simulink model "LinearSimulation"  (R2022b)
settings: Solver=VariableStepAuto  StartTime=0.0  StopTime=10  RelTol=1e-3
undefined symbols (not defined in the file): K, L, T
settings Model: Creator=amirz  LastModifiedBy=amirz

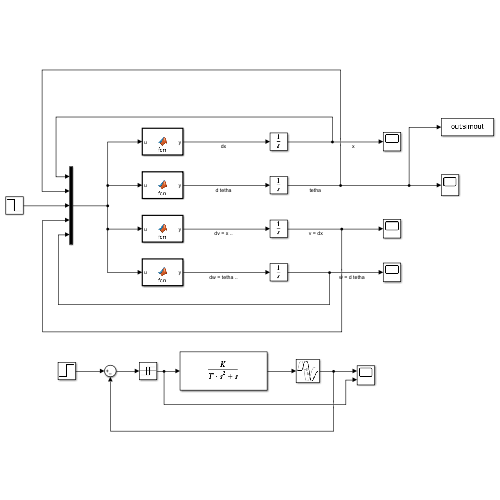
[thumbnail: Simulink's stored preview of the top-level diagram]
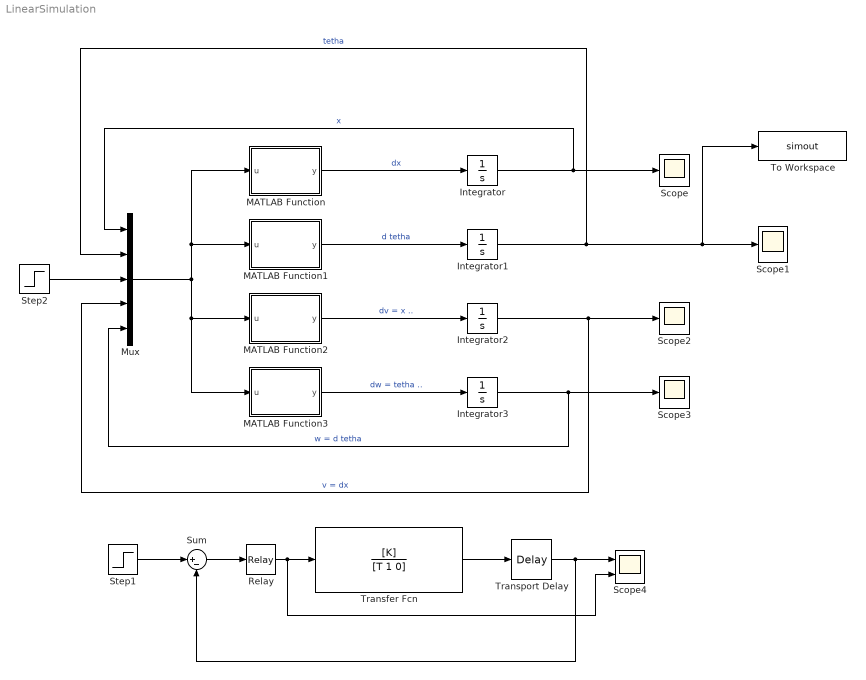
== system LinearSimulation ==
  Integrator{,1..3} (4 alike) : Integrator
  MATLAB Function : MATLAB Function  TreatAsAtomicUnit=on
  MATLAB Function1 : MATLAB Function  TreatAsAtomicUnit=on
  MATLAB Function2 : MATLAB Function  TreatAsAtomicUnit=on
  MATLAB Function3 : MATLAB Function  TreatAsAtomicUnit=on
  Mux : Mux  Inputs=5
  Relay : Relay  OffOutputValue=-1
  Scope{,1..3} (4 alike) : Scope
  Scope4 : Scope  NumInputPorts=2
  Step1 : Step  Time=0  After=0  SampleTime=0
  Step2 : Step  Time=0  After=-1  SampleTime=0
  Sum : Sum  Inputs=|+-
  To Workspace : ToWorkspace  VariableName=simout  SaveFormat=Timeseries  SampleTime=-1
  Transfer Fcn : TransferFcn  Numerator=[K]  Denominator=[T 1 0]
  Transport Delay : TransportDelay  DelayTime=L
  wires:
  Mux/1 -> MATLAB Function2/1(u), MATLAB Function3/1(u), MATLAB Function/1(u), MATLAB Function1/1(u)
  Integrator2/1 -> Scope2/1, Mux/4  "v = dx"
  MATLAB Function1/1(y) -> Integrator1/1  "d tetha"
  MATLAB Function/1(y) -> Integrator/1  "dx"
  Integrator1/1 -> To Workspace/1, Scope1/1, Mux/2  "tetha"
  MATLAB Function2/1(y) -> Integrator2/1  "dv = x .."
  Integrator/1 -> Mux/1, Scope/1  "x"
  MATLAB Function3/1(y) -> Integrator3/1  "dw = tetha .."
  Integrator3/1 -> Mux/5, Scope3/1  "w = d tetha"
  Step2/1 -> Mux/3
  Transfer Fcn/1 -> Transport Delay/1
  Transport Delay/1 -> Scope4/1, Sum/2
  Relay/1 -> Scope4/2, Transfer Fcn/1
  Step1/1 -> Sum/1
  Sum/1 -> Relay/1

== matlab function LinearSimulation/MATLAB Function ==
  data: u input size=[1,5]; y output
function y = fcn(u)
M = 10;
m = 0.3;
l = 0.3;
g = 9.8;
y = u(4);

== matlab function LinearSimulation/MATLAB Function2 ==
  data: u input size=[1,5]; y output
function y = fcn(u)
M = 10;
m = 0.3;
l = 0.3;
g = 9.8;
y = ((u(3) + m*l*u(5)*u(5)*u(2) - m*g*u(2))/(M));

== matlab function LinearSimulation/MATLAB Function3 ==
  data: u input size=[1,5]; y output
function y = fcn(u)
M = 10;
m = 0.3;
l = 0.3;
g = 9.8;
y = ((-u(3) - m*l*u(5)*u(5)*u(2) + M*g*u(2) + m*g*u(2))/(l*M));

== matlab function LinearSimulation/MATLAB Function1 ==
  data: u input size=[1,5]; y output
function y = fcn(u)
M = 10;
m = 0.3;
l = 0.3;
g = 9.8;
y = u(5);
